simulink model "testMeasDataAsBus"  (R2014b)
settings: Solver=ode45  StartTime=0.0  StopTime=max(measData.time)  MaxStep=.005  RelTol=1e-3
settings Model: Creator=fbwk  LastModifiedBy=fbwk
settings DataIOCC: SaveOutput=off  SaveTime=off

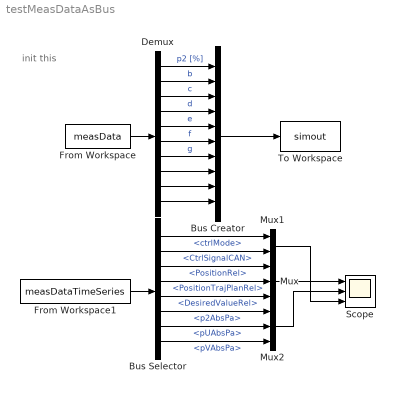
== system testMeasDataAsBus ==
  note: init this
  Bus Creator : BusCreator  Inputs=10
  Bus Selector : BusSelector  OutputSignals=ctrlMode,CtrlSignalCAN,PositionRel,PositionTrajPlanRel,DesiredValueRel,p2AbsPa,pUAbsPa,pVAbsPa
  Demux : Demux  Outputs=10
  From Workspace : FromWorkspace  VariableName=measData  SampleTime=0
  From Workspace1 : FromWorkspace  VariableName=measDataTimeSeries  OutDataTypeStr=Bus: busMeasData  SampleTime=0
  Mux : Mux  Inputs=3
  Mux1 : Mux  Inputs=2
  Mux2 : Mux  Inputs=3
  Scope : Scope  NumInputPorts=3
      settings: ShowLegends=on  YMin=-5~-5~-5  YMax=5~5~5
  To Workspace : ToWorkspace  VariableName=simout  SaveFormat=Timeseries  SampleTime=-1
  wires:
  From Workspace/1 -> Demux/1
  Demux/1 -> Bus Creator/1  "p2 [%]"
  Demux/2 -> Bus Creator/2  "b"
  Demux/3 -> Bus Creator/3  "c"
  Demux/4 -> Bus Creator/4  "d"
  Demux/5 -> Bus Creator/5  "e"
  Demux/6 -> Bus Creator/6  "f"
  Demux/7 -> Bus Creator/7  "g"
  Demux/8 -> Bus Creator/8
  Demux/9 -> Bus Creator/9
  Demux/10 -> Bus Creator/10
  Bus Creator/1 -> To Workspace/1
  From Workspace1/1 -> Bus Selector/1
  Mux/1 -> Scope/1
  Bus Selector/1 -> Mux1/1  "<ctrlMode>"
  Bus Selector/2 -> Mux1/2  "<CtrlSignalCAN>"
  Bus Selector/3 -> Mux/1  "<PositionRel>"
  Bus Selector/4 -> Mux/2  "<PositionTrajPlanRel>"
  Bus Selector/5 -> Mux/3  "<DesiredValueRel>"
  Mux1/1 -> Scope/3
  Bus Selector/6 -> Mux2/1  "<p2AbsPa>"
  Bus Selector/7 -> Mux2/2  "<pUAbsPa>"
  Bus Selector/8 -> Mux2/3  "<pVAbsPa>"
  Mux2/1 -> Scope/2
